simulink model "pruebaGimbal"  (R2018a)
settings: Solver=VariableStepAuto  StartTime=0.0  StopTime=10.0  RelTol=1e-3
settings Model: Creator=Isidro Trabajo  LastModifiedBy=Isidro Trabajo

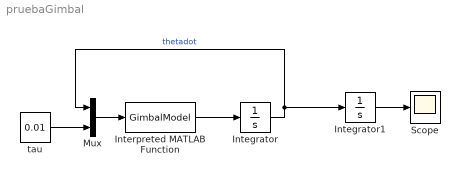
== system pruebaGimbal ==
  Integrator : Integrator
  Integrator1 : Integrator
  Interpreted MATLAB Function : MATLABFcn  MATLABFcn=GimbalModel
  Mux : Mux  Inputs=2
  Scope : Scope
  tau : Constant  Value=0.01
  wires:
  Interpreted MATLAB Function/1 -> Integrator/1
  Integrator/1 -> Integrator1/1, Mux/1  "thetadot"
  Mux/1 -> Interpreted MATLAB Function/1
  tau/1 -> Mux/2
  Integrator1/1 -> Scope/1
